simulink model "Projekt_Dyks_Jozwiak"  (R2013a)
settings: Solver=ode4  SolverMode=SingleTasking  StartTime=0.0  StopTime=30  FixedStep=0.01  RelTol=1e-3  AbsTol=1e-6
InitFcn:
  | mue = 0.0048847; % kg.m
  | J = 0.0016814; % kg.m2
  | g = 9.81; % m/s2
  | 
  | a = (mue*g)/J;
  | 
  | 
  | %%%%%%%%%%%%%% 1 %%
  | A1_1 = 0.2; f1_1 = 15;
  | A2_1 = 0.2; f2_1 = 10;
  | A3_1 = 0.2; f3_1 = 5;
  | %%%%%%%%%%%%%% 2 %%
  | A1_2 = 0.2; f1_2 = 4;
  | A2_2 = 0.2; f2_2 = 12;
  | A3_2 = 0.2; f3_2 = 20;
  | %%%%%%%%%%%%%% 3 %%
  | A1_3 = 0.2; f1_3 = 5;
  | A2_3 = 0.2; f2_3 = 8;
  | A3_3 = 0.2; f3_3 = 10;
  | %%%%%%%%%%%%%% 4 %%
  | A1_4 = 0.2; f1_4 = 20;
  | A2_4 = 0.2; f2_4 = 10;
  | A3_4 = 0.2; f3_4 = 5;
  | 
  | T1 = 0.2;
  | T2 = 0.1;
  | Tf = 0.05;
  | r = 0.1;
  | 
  | b0 = 1;
  | A = [0 1 0;
  |        0 0 1;
  |        0 0 0];
  | b_ = [0; b0; 0];
  | c = [1; 0; 0];
  | 
  | %% Liczenie k
  | w_CL = 5;
  | n=2;
  | k = zeros(n,1);
  | for i = 1:n
  |     k(i) = ((factorial(n))/(factorial(n-i+1)*factorial(i-1)))*w_CL^(n-i+1);
  | end
  | 
  | k_r = [k(2); 1];
  | 
  | %% Liczenie l
  | k_ESO = 50;
  | l = zeros(n+1,1);
  | 
  | for i = 1:n+1
  |     l(i) = (factorial(n+1)/(factorial(n-i+1)*factorial(i)))*(k_ESO)^(i);
  | end
  | 
  | %% W ARTYKULE MADONSKI K,L ODPOWIADA L I B W ARTYKULE JIN H.
  | l1 = k(2);
  | l2 = k(1);
  | 
  | B1 = l(1);
  | B2 = l(2);
  | B3 = l(3);
  | 
  | %% WYZNACZENIE PARAMETRÓW:
  | Kc = (B2 * l2 + B3 * l1)/(b0*(B1 * l1 + B2 + l2));
  | tau_i = (B2 * l2 + B3 * l1)/(B3 * l2);
  | tau_d = (B1 * l2 + B2 * l1 + B3)/(B2 * l2 + B3 * l1);
  | wl = sqrt(B1 * l1 + B2 + l2);
  | zeta_l = (B1 + l1)/(2*sqrt(B1 * l1 + B2 + l2));
  | %% Wzmocnienia regulatora CPID:
  | Kp = Kc;
  | Ki = Kc/tau_i;
  | Kd = Kc * tau_d;
undefined symbols (not defined in the file): RTDAC4PCIBaseAddress
libraries: simulink x2
settings Model: SimulationMode=external  ExtModeTrigDuration=50000  ExtModeTrigLevel=0.400000  Creator=jims  LastModifiedBy=Pracownik
settings DataIOCC: ExternalInput=[]  InitialState=[]  LimitDataPoints=off  MaxDataPoints=5000  SignalLoggingSaveFormat=ModelDataLogs  SaveOutput=off  SaveTime=off  SignalLoggingName=sigsOut
settings OptimizationCC: BooleanDataType=off  ExpressionDepthLimit=2147483647  InitFltsAndDblsToZero=on
settings DebuggingCC: SaveWithParameterizedLinksMsg=none  SignalResolutionControl=TryResolveAllWithWarning  SolverPrmCheckMsg=none  MultiTaskDSMMsg=warning  MultiTaskCondExecSysMsg=none  IntegerOverflowMsg=none  FcnCallInpInsideContextMsg=UseLocalSettings  StrictBusMsg=None
settings HardwareCC: ProdIntDivRoundTo=Zero  ProdEndianess=LittleEndian  ProdHWDeviceType=Generic->32-bit x86 compatible
settings RTWCC: SystemTargetFile=rtwin.tlc  TemplateMakefile=rtwin.tmf  Description=Real-Time Windows Target  ProcessScript=rtwin_make_rtw_hook  IncludeERTFirstTime=on  RTWCompilerOptimization=On
settings CodeAppCC: MaxIdLength=95
settings RTWinTargetCC: TargetLibSuffix=_rtwin.lib  TargetPreCompLibLocation=C:\Program Files\MATLAB\R2013a\toolbox\rtw\targets\rtwin\lib\win64  CodeReplacementLibrary=ANSI_C  RTWinDir=C:/PROGRA~1/MATLAB/R2013a/toolbox/rtw/targets/rtwin  TargetArch=win64

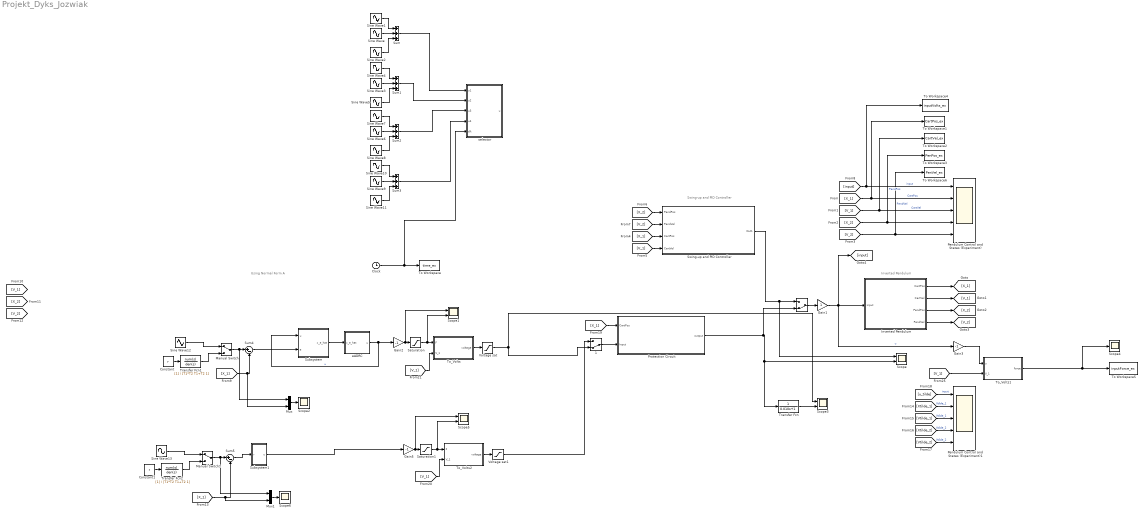
== system Projekt_Dyks_Jozwiak ==
  note: Using Normal Form A
  note: Inverted Pendulum
  note: Swing-up and PID Controller
  " " : ManualSwitch  CurrentSetting=0
  " 1" : ManualSwitch  CurrentSetting=0
  Clock : Clock
  Constant : Constant  Value=r
  Constant1 : Constant  Value=r
  Gain1 : Gain
  Gain2 : Gain  Gain=-1
  Gain3 : Gain  Gain=-1
  Gain5 : Gain  Gain=-1
  Inverted Pendulum : Subsystem
  Manual Switch : ManualSwitch
  Manual Switch1 : ManualSwitch
  Mux : Mux  Inputs=2
  Mux1 : Mux  Inputs=2
  Pendulum Control and States (Experiment) : Scope  NumInputPorts=5
      settings: TimeRange=7  YMin=-0.125~-0.125~-0.125~-3.5~-175000  YMax=0.15~0.125~0.125~3.5~175000  SaveName=P1_Data  MaxDataPoints=50000
  Pendulum Control and States (Experiment)1 : Scope  NumInputPorts=5
      settings: TimeRange=10  YMin=-1~-4~-7.5~-0.125~-0.25  YMax=1~4~7.5~0.075~0.2  SaveName=P1_Data1  MaxDataPoints=50000
  Protection Circuit : Subsystem
  Saturation : Saturate  UpperLimit=500  LowerLimit=-500
  Saturation1 : Saturate  UpperLimit=500  LowerLimit=-500
  Scope{,1,3,5} (4 alike) : Scope  NumInputPorts=2
      Scope settings: YMin=-5~-5  YMax=5~5
      Scope1 settings: YMin=-5~-5  YMax=5~5  SaveName=ScopeData2
      Scope3 settings: YMin=-0.3~-0.225  YMax=0.275~0.15  SaveName=ScopeData5
      Scope5 settings: YMin=-5~-5  YMax=5~5  SaveName=ScopeData6
  Scope2 : Scope
      settings: YMin=-0.11  YMax=0.11  SaveName=ScopeData3
  Scope4 : Scope
      settings: SaveName=ScopeData4
  Scope6 : Scope
      settings: YMin=-0.11  YMax=0.11  SaveName=ScopeData7
  Sine Wave : Sin  Amplitude=A2_1  Frequency=f2_1  SampleTime=0
  Sine Wave1 : Sin  Amplitude=A1_1  Frequency=f1_1  SampleTime=0
  Sine Wave10 : Sin  Amplitude=A1_4  Frequency=f1_4  SampleTime=0
  Sine Wave11 : Sin  Amplitude=A3_4  Frequency=f3_4  SampleTime=0
  Sine Wave12 : Sin  Amplitude=r  SampleTime=0
  Sine Wave13 : Sin  Amplitude=r  SampleTime=0
  Sine Wave2 : Sin  Amplitude=A3_1  Frequency=f3_1  SampleTime=0
  Sine Wave3 : Sin  Amplitude=A2_2  Frequency=f2_2  SampleTime=0
  Sine Wave4 : Sin  Amplitude=A1_2  Frequency=f1_2  SampleTime=0
  Sine Wave5 : Sin  Amplitude=A3_2  Frequency=f3_2  SampleTime=0
  Sine Wave6 : Sin  Amplitude=A2_3  Frequency=f2_3  SampleTime=0
  Sine Wave7 : Sin  Amplitude=A1_3  Frequency=f1_3  SampleTime=0
  Sine Wave8 : Sin  Amplitude=A3_3  Frequency=f3_3  SampleTime=0
  Sine Wave9 : Sin  Amplitude=A2_4  Frequency=f2_4  SampleTime=0
  Subsystem : Subsystem
  Subsystem1 : Subsystem
  Sum{,1..3} (4 alike) : Sum  Inputs=+++
  Sum4 : Sum  Inputs=|+-
  Sum5 : Sum  Inputs=|+-
  Swing-up and PID Controller : Subsystem
  To Workspace : ToWorkspace  VariableName=time_ex  SampleTime=-1
  To Workspace1 : ToWorkspace  VariableName=CartPos_ex  SampleTime=-1
  To Workspace2 : ToWorkspace  VariableName=CartVel_ex  SampleTime=-1
  To Workspace3 : ToWorkspace  VariableName=PenPos_ex  SampleTime=-1
  To Workspace4 : ToWorkspace  VariableName=inputVolts_ex  SampleTime=-1
  To Workspace5 : ToWorkspace  VariableName=inputForce_ex  SampleTime=-1
  To Workspace6 : ToWorkspace  VariableName=PenVel_ex  SampleTime=-1
  To_Volts : MATLAB Function  TreatAsAtomicUnit=on
  To_Volts1 : MATLAB Function  TreatAsAtomicUnit=on
  To_Volts2 : MATLAB Function  TreatAsAtomicUnit=on
  Transfer Fcn : TransferFcn  Denominator=[0.010 1]
  Transfer Fcn1 : TransferFcn  Denominator=[T1*T2 T1+T2 1]
  Transfer Fcn2 : TransferFcn  Denominator=[T1*T2 T1+T2 1]
  Voltage sat : Saturate  UpperLimit=0.6  LowerLimit=-0.6
  Voltage sat1 : Saturate  UpperLimit=0.6  LowerLimit=-0.6
  "eADRC " : Subsystem
  selector : MATLAB Function  TreatAsAtomicUnit=on
  wires:
  [V_2] -> To Workspace6/1, Pendulum Control and States (Experiment)/5  "PendVel"
  [X_2] -> To Workspace3/1, Pendulum Control and States (Experiment)/4  "PendPos"
  [V_1] -> To Workspace2/1, Pendulum Control and States (Experiment)/3  "CartVel"
  [X_1] -> To Workspace1/1, Pendulum Control and States (Experiment)/2  "CartPos"
  Inverted Pendulum/1(CartPos) -> [X_1]
  Inverted Pendulum/2(CartVel) -> [V_1]
  Inverted Pendulum/3(PendPos) -> [X_2]
  Inverted Pendulum/4(PendVel) -> [V_2]
  [X_2] -> Swing-up and PID Controller/1(PendPos)
  [V_2] -> Swing-up and PID Controller/2(PendVel)
  [X_1] -> Swing-up and PID Controller/3(CartPos)
  [V_1] -> Swing-up and PID Controller/4(CartVel)
  [input] -> To Workspace4/1, Pendulum Control and States (Experiment)/1  "input"
  Swing-up and PID Controller/1(Out1) -> Scope/1, " "/1
  "eADRC "/1("u ") -> Subsystem/1("u "), Gain2/1  "u"
  [Vtilde_2] -> Pendulum Control and States (Experiment)1/5  "Vtilde_2"
  [Xtilde_2] -> Pendulum Control and States (Experiment)1/4  "Xtilde_2"
  [Vtilde_1] -> Pendulum Control and States (Experiment)1/3  "Vtilde_1"
  [Xtilde_1] -> Pendulum Control and States (Experiment)1/2  "Xtilde_1"
  [u_tilde] -> Pendulum Control and States (Experiment)1/1  "input"
  Gain2/1 -> Saturation/1, Scope1/1
  [X_1] -> Protection Circuit/1(CartPos)
  Saturation/1 -> Scope1/2, To_Volts/1(F)
  [V_1] -> To_Volts/2(V_1)
  [X_1] -> Mux/2, Sum4/2
  " "/1 -> Gain1/1
  To_Volts/1(voltage) -> Voltage sat/1
  Transfer Fcn/1 -> Scope3/2
  Clock/1 -> selector/5(clk), To Workspace/1
  Protection Circuit/1(output) -> " "/2, Transfer Fcn/1, Scope/2
  Voltage sat/1 -> " 1"/2, Scope3/1
  " 1"/1 -> Protection Circuit/2(Input)
  Gain1/1 -> Gain3/1, Inverted Pendulum/1(input), [input]  "u"
  To_Volts1/1(force) -> Scope4/1, To Workspace5/1
  Gain3/1 -> To_Volts1/1(u)
  [V_1] -> To_Volts1/2(V_1)
  Sine Wave1/1 -> Sum/1
  Sine Wave/1 -> Sum/2
  Sine Wave2/1 -> Sum/3
  Sum/1 -> selector/1(u1)
  Sum1/1 -> selector/2(u2)
  Sum2/1 -> selector/3(u3)
  Sum3/1 -> selector/4(u4)
  Sine Wave4/1 -> Sum1/1
  Sine Wave3/1 -> Sum1/2
  Sine Wave5/1 -> Sum1/3
  Sine Wave7/1 -> Sum2/1
  Sine Wave6/1 -> Sum2/2
  Sine Wave8/1 -> Sum2/3
  Sine Wave10/1 -> Sum3/1
  Sine Wave9/1 -> Sum3/2
  Sine Wave11/1 -> Sum3/3
  Subsystem/1("x_e_hat ") -> "eADRC "/1("x_e_hat ")
  Constant/1 -> Transfer Fcn1/1
  Sine Wave12/1 -> Manual Switch/1
  Transfer Fcn1/1 -> Manual Switch/2
  Manual Switch/1 -> Mux/1, Sum4/1
  Sum4/1 -> Subsystem/2("e ")
  Mux/1 -> Scope2/1
  Constant1/1 -> Transfer Fcn2/1
  Sine Wave13/1 -> Manual Switch1/1
  Transfer Fcn2/1 -> Manual Switch1/2
  Manual Switch1/1 -> Mux1/1, Sum5/1
  Sum5/1 -> Subsystem1/1(r)
  [X_1] -> Mux1/2, Sum5/2
  Gain5/1 -> Saturation1/1, Scope5/1
  Saturation1/1 -> Scope5/2, To_Volts2/1(F)
  [V_1] -> To_Volts2/2(V_1)
  To_Volts2/1(voltage) -> Voltage sat1/1
  Subsystem1/1("u ") -> Gain5/1
  Voltage sat1/1 -> " 1"/1
  Mux1/1 -> Scope6/1

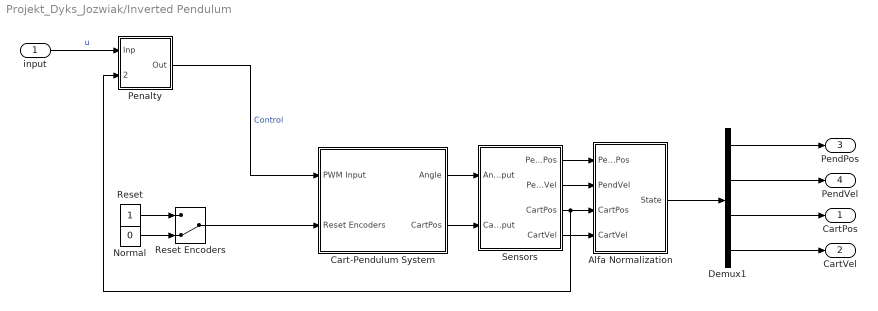
== system Projekt_Dyks_Jozwiak/Inverted Pendulum ==
  input : Inport
  Alfa Normalization : Subsystem  mask(Choose mode:){pos=Inverted Pendulum}
      mask prompts: pos "Choose mode:"
      mask TypeOptions pos: Inverted Pendulum | Crane Controller
  Cart-Pendulum System : Subsystem  mask{BaseAddress=RTDAC4PCIBaseAddress, T0=0.01}
      mask prompts: BaseAddress "Base Address:"; T0 "Sampling Period:"
      mask Display: plot( [0.725 0.725], [1.05 0.375], 0.725+0.05*sin([0:0.5:7]), 0.325+0.05*cos([0:0.5:7]), [-0.3 -0.3], [-0.3 -0.3], [1.8 1.8], [1.8 1.8], [0.1 1.4], [0.95 0.95], [0.1 1.4], [0.92 0.92], [0.65 0.8], [1 1], [0.65 0.8], [1.1 1.1], [0.65 0.65], [1.1 1], [0.8 0.8], [1 1.1] )
  Demux1 : Demux
  Normal : Constant  Value=0
  Penalty : Subsystem
  Reset : Constant
  Reset Encoders : ManualSwitch  CurrentSetting=0
  Sensors : Subsystem  mask(PENDULUM Output){T0=0.01}
      mask prompts: T0 "Sample Time"
      mask help: PCL-812 PG Device Driver
  CartPos : Outport
  CartVel : Outport  Port=2
  PendPos : Outport  Port=3
  PendVel : Outport  Port=4
  wires:
  Penalty/1(Out) -> Cart-Pendulum System/1(PWM Input)  "Control"
  Cart-Pendulum System/2(CartPos) -> Sensors/2(CartPosInput)
  Cart-Pendulum System/1(Angle) -> Sensors/1(AngleInput)
  Sensors/1(PendPos) -> Alfa Normalization/1(PendPos)
  Alfa Normalization/1(State) -> Demux1/1
  Sensors/2(PendVel) -> Alfa Normalization/2(PendVel)
  Reset/1 -> Reset Encoders/1
  Sensors/4(CartVel) -> Alfa Normalization/4(CartVel)
  Normal/1 -> Reset Encoders/2
  Reset Encoders/1 -> Cart-Pendulum System/2(Reset Encoders)
  Sensors/3(CartPos) -> Penalty/2(CartPos), Alfa Normalization/3(CartPos)
  Demux1/2 -> PendVel/1
  Demux1/1 -> PendPos/1
  Demux1/4 -> CartVel/1
  Demux1/3 -> CartPos/1
  input/1 -> Penalty/1(Inp)  "u"

== system Projekt_Dyks_Jozwiak/Protection Circuit ==
  CartPos : Inport
  Input : Inport  Port=2
  4 : Switch  SaturateOnIntegerOverflow=on  InputSameDT=on
  Rail limiter : MATLAB Function  TreatAsAtomicUnit=on
  Saturation1 : Saturate  UpperLimit=1  LowerLimit=-1
  Sign : Signum
  output : Outport
  wires:
  Rail limiter/1(logic) -> 4/2
  Sign/1 -> 4/1  "max"
  Input/1 -> 4/3
  CartPos/1 -> Rail limiter/1(CartPos), Sign/1
  4/1 -> Saturation1/1
  Saturation1/1 -> output/1

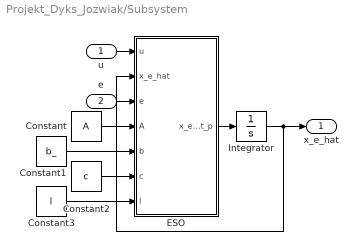
== system Projekt_Dyks_Jozwiak/Subsystem ==
  "u " : Inport
  "e " : Inport  Port=2
  Constant : Constant  Value=A
  Constant1 : Constant  Value=b_
  Constant2 : Constant  Value=c
  Constant3 : Constant  Value=l
  "ESO " : MATLAB Function  TreatAsAtomicUnit=on
  Integrator : Integrator  InitialCondition=[0; 0; 0]
  "x_e_hat " : Outport
  wires:
  Constant2/1 -> "ESO "/6(c)
  Constant/1 -> "ESO "/4(A)
  "ESO "/1(x_e_hat_p) -> Integrator/1
  Integrator/1 -> "x_e_hat "/1, "ESO "/2(x_e_hat)
  "u "/1 -> "ESO "/1(u)
  "e "/1 -> "ESO "/3(e)
  Constant3/1 -> "ESO "/7(l)
  Constant1/1 -> "ESO "/5(b)

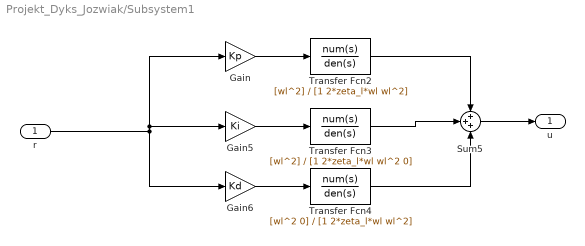
== system Projekt_Dyks_Jozwiak/Subsystem1 ==
  r : Inport
  Gain : Gain  Gain=Kp
  Gain5 : Gain  Gain=Ki
  Gain6 : Gain  Gain=Kd
  Sum5 : Sum  Inputs=+++
  Transfer Fcn2 : TransferFcn  Numerator=[wl^2]  Denominator=[1 2*zeta_l*wl wl^2]
  Transfer Fcn3 : TransferFcn  Numerator=[wl^2]  Denominator=[1 2*zeta_l*wl wl^2 0]
  Transfer Fcn4 : TransferFcn  Numerator=[wl^2 0]  Denominator=[1 2*zeta_l*wl wl^2]
  "u " : Outport
  wires:
  Transfer Fcn3/1 -> Sum5/2
  r/1 -> Gain/1, Gain5/1, Gain6/1
  Transfer Fcn4/1 -> Sum5/3
  Sum5/1 -> "u "/1
  Gain5/1 -> Transfer Fcn3/1
  Transfer Fcn2/1 -> Sum5/1
  Gain6/1 -> Transfer Fcn4/1
  Gain/1 -> Transfer Fcn2/1

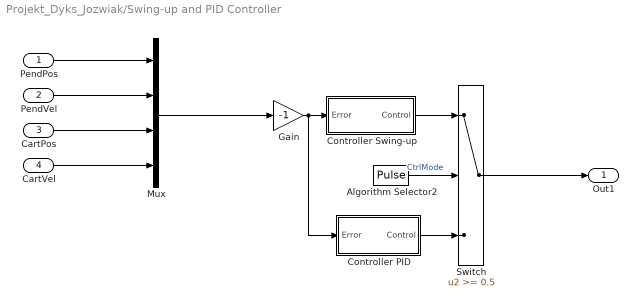
== system Projekt_Dyks_Jozwiak/Swing-up and PID Controller ==
  PendPos : Inport
  PendVel : Inport  Port=2
  CartPos : Inport  Port=3
  CartVel : Inport  Port=4
  Algorithm Selector2 : DiscretePulseGenerator  PulseType=Time based  Period=60  PulseWidth=85  SampleTime=0.01
  Controller PID : Subsystem  mask{Cart_PID=[ -0.8 -0.0 -0.05], Pend_PID=[-1 0 -0.0 ], Umax=0.5, zone=1.3, Friction=0.05, T0=0.01}
      mask prompts: Cart_PID "Cart PID parameters [Kp, Ki, Kd]:"; Pend_PID "Pendulum PID parameters [Kp, Ki, Kd]:"; Umax "Maximum control value:"; zone "Stabilisation zone [rad]:"; Friction "Friction compensation:"; T0 "Sample time:"
  Controller Swing-up : Subsystem
  Gain : Gain  Gain=-1
  Mux : Mux
  Switch : Switch  Threshold=0.5  SaturateOnIntegerOverflow=on  InputSameDT=on
  Out1 : Outport
  wires:
  Controller Swing-up/1(Control) -> Switch/1
  Algorithm Selector2/1 -> Switch/2  "CtrlMode"
  Gain/1 -> Controller Swing-up/1(Error), Controller PID/1(Error)
  Controller PID/1(Control) -> Switch/3
  Switch/1 -> Out1/1
  PendVel/1 -> Mux/2
  PendPos/1 -> Mux/1
  CartPos/1 -> Mux/3
  CartVel/1 -> Mux/4
  Mux/1 -> Gain/1

== system Projekt_Dyks_Jozwiak/eADRC  ==
  "x_e_hat " : Inport
  Constant : Constant  Value=b0
  Constant1 : Constant  Value=k
  MATLAB Function : MATLAB Function  TreatAsAtomicUnit=on
  "u " : Outport
  wires:
  Constant/1 -> MATLAB Function/1(b0)
  Constant1/1 -> MATLAB Function/2(k)
  MATLAB Function/1(u) -> "u "/1
  "x_e_hat "/1 -> MATLAB Function/3(x_e_hat)

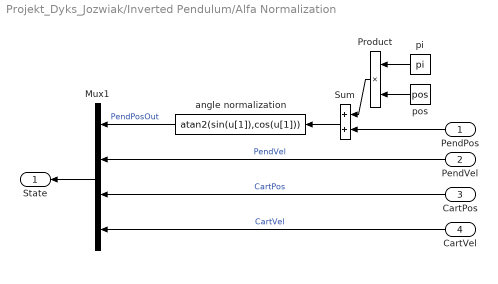
== system Projekt_Dyks_Jozwiak/Inverted Pendulum/Alfa Normalization ==
  PendPos : Inport
  PendVel : Inport  Port=2
  CartPos : Inport  Port=3
  CartVel : Inport  Port=4
  Mux1 : Mux
  Product : Product  SaturateOnIntegerOverflow=on  InputSameDT=on  OutDataTypeStr=Inherit: Same as first input
  Sum : Sum  SaturateOnIntegerOverflow=on  InputSameDT=on  OutDataTypeStr=Inherit: Same as first input
  angle normalization : Fcn  Expr=atan2(sin(u[1]),cos(u[1]))
  pi : Constant  Value=pi
  pos : Constant  Value=pos
  State : Outport  InitialOutput=0
  wires:
  angle normalization/1 -> Mux1/1  "PendPosOut"
  PendVel/1 -> Mux1/2  "PendVel"
  CartVel/1 -> Mux1/4  "CartVel"
  CartPos/1 -> Mux1/3  "CartPos"
  Mux1/1 -> State/1
  Sum/1 -> angle normalization/1
  PendPos/1 -> Sum/2
  pi/1 -> Product/1
  pos/1 -> Product/2
  Product/1 -> Sum/1

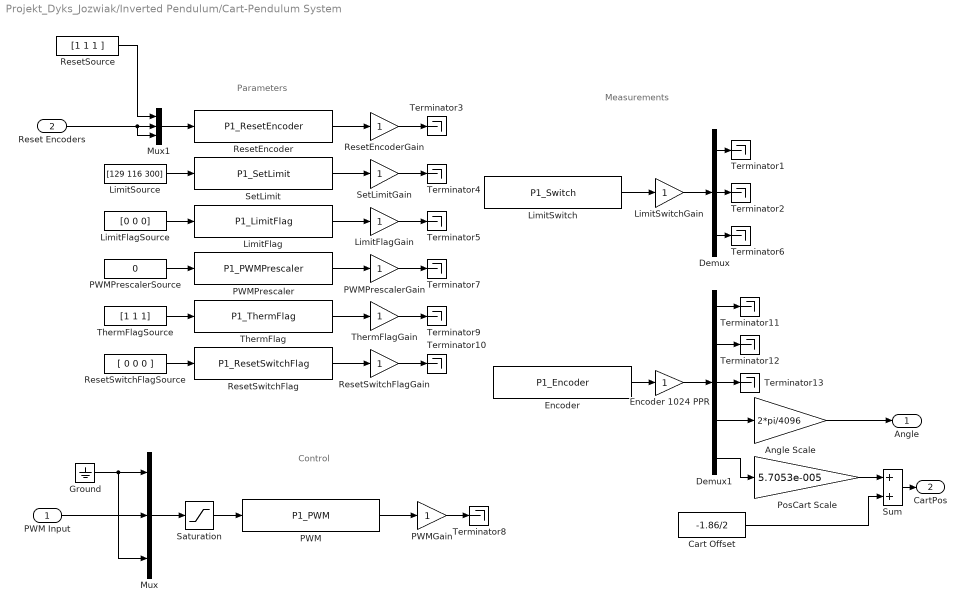
== system Projekt_Dyks_Jozwiak/Inverted Pendulum/Cart-Pendulum System ==
  note: Measurements
  note: Control
  note: Parameters
  PWM Input : Inport
  Reset Encoders : Inport  Port=2
  Angle Scale : Gain  Gain=2*pi/4096  OutDataTypeStr=Inherit: Same as input  ParamDataTypeStr=Inherit: Same as input
  Cart Offset : Constant  Value=-1.86/2
  Demux : Demux  Outputs=3
  Demux1 : Demux  Outputs=5
  Encoder : S-Function  FunctionName=P1_Encoder  Parameters=BaseAddress, T0  EnableBusSupport=off
  Encoder 1024 PPR : Gain  SaturateOnIntegerOverflow=on  OutDataTypeStr=Inherit: Same as input  ParamDataTypeStr=Inherit: Same as input
  Ground : Ground
  LimitFlag : S-Function  FunctionName=P1_LimitFlag  Parameters=BaseAddress, T0  EnableBusSupport=off
  LimitFlagGain : Gain  SaturateOnIntegerOverflow=on  OutDataTypeStr=Inherit: Same as input  ParamDataTypeStr=Inherit: Same as input
  LimitFlagSource : Constant  Value=[0 0 0]
  LimitSource : Constant  Value=[129 116 300]
  LimitSwitch : S-Function  FunctionName=P1_Switch  Parameters=BaseAddress, T0  EnableBusSupport=off
  LimitSwitchGain : Gain  SaturateOnIntegerOverflow=on  OutDataTypeStr=Inherit: Same as input  ParamDataTypeStr=Inherit: Same as input
  Mux : Mux  Inputs=3
  Mux1 : Mux  Inputs=[3 1 1]
  PWM : S-Function  FunctionName=P1_PWM  Parameters=BaseAddress, T0  EnableBusSupport=off
  PWMGain : Gain  SaturateOnIntegerOverflow=on  OutDataTypeStr=Inherit: Same as input  ParamDataTypeStr=Inherit: Same as input
  PWMPrescaler : S-Function  FunctionName=P1_PWMPrescaler  Parameters=BaseAddress, T0  EnableBusSupport=off
  PWMPrescalerGain : Gain  SaturateOnIntegerOverflow=on  OutDataTypeStr=Inherit: Same as input  ParamDataTypeStr=Inherit: Same as input
  PWMPrescalerSource : Constant  Value=0
  PosCart Scale : Gain  Gain=5.7053e-005  OutDataTypeStr=Inherit: Same as input  ParamDataTypeStr=Inherit: Same as input
  ResetEncoder : S-Function  FunctionName=P1_ResetEncoder  Parameters=BaseAddress, T0  EnableBusSupport=off
  ResetEncoderGain : Gain  SaturateOnIntegerOverflow=on  OutDataTypeStr=Inherit: Same as input  ParamDataTypeStr=Inherit: Same as input
  ResetSource : Constant  Value=[1 1 1 ]
  "ResetSwitchFlag " : S-Function  FunctionName=P1_ResetSwitchFlag  Parameters=BaseAddress, T0  EnableBusSupport=off
  ResetSwitchFlagGain : Gain  SaturateOnIntegerOverflow=on  OutDataTypeStr=Inherit: Same as input  ParamDataTypeStr=Inherit: Same as input
  ResetSwitchFlagSource : Constant  Value=[ 0 0 0 ]
  Saturation : Saturate  UpperLimit=1  LowerLimit=-1
  SetLimit : S-Function  FunctionName=P1_SetLimit  Parameters=BaseAddress, T0  EnableBusSupport=off
  SetLimitGain : Gain  SaturateOnIntegerOverflow=on  OutDataTypeStr=Inherit: Same as input  ParamDataTypeStr=Inherit: Same as input
  Sum : Sum  SaturateOnIntegerOverflow=on  InputSameDT=on  OutDataTypeStr=Inherit: Same as first input
  Terminator{1..13} (13 alike) : Terminator
  "ThermFlag " : S-Function  FunctionName=P1_ThermFlag  Parameters=BaseAddress, T0  EnableBusSupport=off
  ThermFlagGain : Gain  SaturateOnIntegerOverflow=on  OutDataTypeStr=Inherit: Same as input  ParamDataTypeStr=Inherit: Same as input
  ThermFlagSource : Constant  Value=[1 1 1]
  Angle : Outport
  CartPos : Outport  Port=2
  wires:
  Demux1/1 -> Terminator11/1
  Demux1/2 -> Terminator12/1
  Demux1/3 -> Terminator13/1
  Demux1/4 -> Angle Scale/1
  Demux1/5 -> PosCart Scale/1
  Angle Scale/1 -> Angle/1
  Demux/3 -> Terminator6/1
  Demux/2 -> Terminator2/1
  Demux/1 -> Terminator1/1
  LimitSwitchGain/1 -> Demux/1
  LimitSwitch/1 -> LimitSwitchGain/1
  Ground/1 -> Mux/1, Mux/3
  PWM Input/1 -> Mux/2
  ResetSwitchFlagGain/1 -> Terminator10/1
  ThermFlagGain/1 -> Terminator9/1
  PWMPrescalerGain/1 -> Terminator7/1
  LimitFlagGain/1 -> Terminator5/1
  SetLimitGain/1 -> Terminator4/1
  ResetEncoderGain/1 -> Terminator3/1
  ResetSwitchFlagSource/1 -> "ResetSwitchFlag "/1
  ThermFlagSource/1 -> "ThermFlag "/1
  PWMPrescalerSource/1 -> PWMPrescaler/1
  LimitFlagSource/1 -> LimitFlag/1
  LimitSource/1 -> SetLimit/1
  "ResetSwitchFlag "/1 -> ResetSwitchFlagGain/1
  "ThermFlag "/1 -> ThermFlagGain/1
  PWMPrescaler/1 -> PWMPrescalerGain/1
  LimitFlag/1 -> LimitFlagGain/1
  SetLimit/1 -> SetLimitGain/1
  ResetEncoder/1 -> ResetEncoderGain/1
  PWMGain/1 -> Terminator8/1
  PWM/1 -> PWMGain/1
  Mux/1 -> Saturation/1
  Saturation/1 -> PWM/1
  Encoder/1 -> Encoder 1024 PPR/1
  Encoder 1024 PPR/1 -> Demux1/1
  Mux1/1 -> ResetEncoder/1
  ResetSource/1 -> Mux1/1
  Reset Encoders/1 -> Mux1/2, Mux1/3
  PosCart Scale/1 -> Sum/1
  Sum/1 -> CartPos/1
  Cart Offset/1 -> Sum/2

== system Projekt_Dyks_Jozwiak/Inverted Pendulum/Penalty ==
  Inp : Inport
  CartPos : Inport  Port=2
  CtrlSat : Saturate  UpperLimit=1  LowerLimit=-1
  Fcn : Fcn  Expr=(u>=0.8)*(10*(u-0.8))^3 + (u<=-0.8)*(10*(u+0.8))^3
  Sum : Sum  Inputs=|++  SaturateOnIntegerOverflow=on  InputSameDT=on  OutDataTypeStr=Inherit: Same as first input
  Out : Outport
  wires:
  Inp/1 -> Out/1, Sum/1
  CartPos/1 -> Fcn/1
  Sum/1 -> CtrlSat/1
  Fcn/1 -> Sum/2

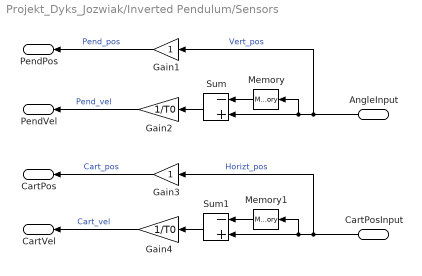
== system Projekt_Dyks_Jozwiak/Inverted Pendulum/Sensors ==
  AngleInput : Inport
  CartPosInput : Inport  Port=2
  Gain1 : Gain  SaturateOnIntegerOverflow=on  OutDataTypeStr=Inherit: Same as input  ParamDataTypeStr=Inherit: Same as input
  Gain2 : Gain  Gain=1/T0  SaturateOnIntegerOverflow=on  OutDataTypeStr=Inherit: Same as input  ParamDataTypeStr=Inherit: Same as input
  Gain3 : Gain  SaturateOnIntegerOverflow=on  OutDataTypeStr=Inherit: Same as input  ParamDataTypeStr=Inherit: Same as input
  Gain4 : Gain  Gain=1/T0  SaturateOnIntegerOverflow=on  OutDataTypeStr=Inherit: Same as input  ParamDataTypeStr=Inherit: Same as input
  Memory : Memory
  Memory1 : Memory
  Sum : Sum  Inputs=-+  SaturateOnIntegerOverflow=on  InputSameDT=on  OutDataTypeStr=Inherit: Same as first input
  Sum1 : Sum  Inputs=-+  SaturateOnIntegerOverflow=on  InputSameDT=on  OutDataTypeStr=Inherit: Same as first input
  PendPos : Outport  InitialOutput=0
  PendVel : Outport  Port=2  InitialOutput=0
  CartPos : Outport  Port=3  InitialOutput=0
  CartVel : Outport  Port=4  InitialOutput=0
  wires:
  Gain4/1 -> CartVel/1  "Cart_vel"
  Sum1/1 -> Gain4/1
  Memory1/1 -> Sum1/1
  Sum/1 -> Gain2/1
  Memory/1 -> Sum/1
  CartPosInput/1 -> Memory1/1, Sum1/2, Gain3/1  "Horizt_pos"
  AngleInput/1 -> Memory/1, Sum/2, Gain1/1  "Vert_pos"
  Gain2/1 -> PendVel/1  "Pend_vel"
  Gain1/1 -> PendPos/1  "Pend_pos"
  Gain3/1 -> CartPos/1  "Cart_pos"

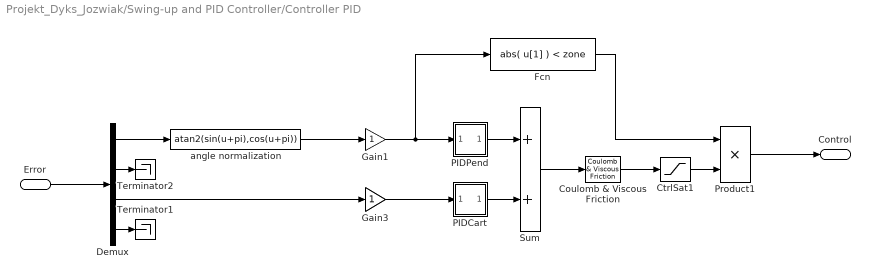
== system Projekt_Dyks_Jozwiak/Swing-up and PID Controller/Controller PID ==
  Error : Inport
  Coulomb & Viscous Friction : simulink/Discontinuities/Coulomb & Viscous Friction  offset=Friction  gain=1
  CtrlSat1 : Saturate  UpperLimit=Umax  LowerLimit=-Umax
  Demux : Demux
  Fcn : Fcn  Expr=abs( u[1] ) < zone
  Gain1 : Gain  SaturateOnIntegerOverflow=on  OutDataTypeStr=Inherit: Same as input  ParamDataTypeStr=Inherit: Same as input
  Gain3 : Gain  SaturateOnIntegerOverflow=on  OutDataTypeStr=Inherit: Same as input  ParamDataTypeStr=Inherit: Same as input
  PIDCart : Subsystem  mask(PID(2) Controller){P=Cart_PID(1), I=Cart_PID(2), D=Cart_PID(3), T0=T0}
      mask prompts: P "Proportional:"; I "Integral:"; D "Derivative:"; T0 "Sample Time:"
      mask help:
      | Enter Proportional(P), Integral(I), and Derivative(D) and divisor (N) terms.
      | P+I/s+Ds/(1/Ns+1)
      mask Help: This block implements a PID controller where parameters are entered for the Proportional, Integral and Derivative and divisor terms. Unmask this block to see how it works. The derivative term is implemented using an s/(s/N +1)  transfer function block. Making N large can create a "stiff" system.
      mask Display: disp('PID')
  PIDPend : Subsystem  mask(PID(2) Controller){P=Pend_PID(1), I=Pend_PID(2), D=Pend_PID(3), T0=T0}
      mask prompts: P "Proportional:"; I "Integral:"; D "Derivative:"; T0 "Sample Time:"
      mask help:
      | Enter Proportional(P), Integral(I), and Derivative(D) and divisor (N) terms.
      | P+I/s+Ds/(1/Ns+1)
      mask Help: This block implements a PID controller where parameters are entered for the Proportional, Integral and Derivative and divisor terms. Unmask this block to see how it works. The derivative term is implemented using an s/(s/N +1)  transfer function block. Making N large can create a "stiff" system.
      mask Display: disp('PID')
  Product1 : Product  SaturateOnIntegerOverflow=on  InputSameDT=on  OutDataTypeStr=Inherit: Same as first input
  Sum : Sum  SaturateOnIntegerOverflow=on  InputSameDT=on  OutDataTypeStr=Inherit: Same as first input
  Terminator1 : Terminator
  Terminator2 : Terminator
  angle normalization : Fcn  Expr=atan2(sin(u+pi),cos(u+pi))
  Control : Outport  InitialOutput=0
  wires:
  Demux/4 -> Terminator1/1
  Demux/3 -> Gain3/1
  Demux/2 -> Terminator2/1
  Error/1 -> Demux/1
  Demux/1 -> angle normalization/1
  Gain1/1 -> Fcn/1, PIDPend/1(In_1)
  PIDPend/1(Out_1) -> Sum/1
  Sum/1 -> Coulomb & Viscous Friction/1
  Coulomb & Viscous Friction/1 -> CtrlSat1/1
  CtrlSat1/1 -> Product1/2
  Fcn/1 -> Product1/1
  Product1/1 -> Control/1
  Gain3/1 -> PIDCart/1(In_1)
  PIDCart/1(Out_1) -> Sum/2
  angle normalization/1 -> Gain1/1

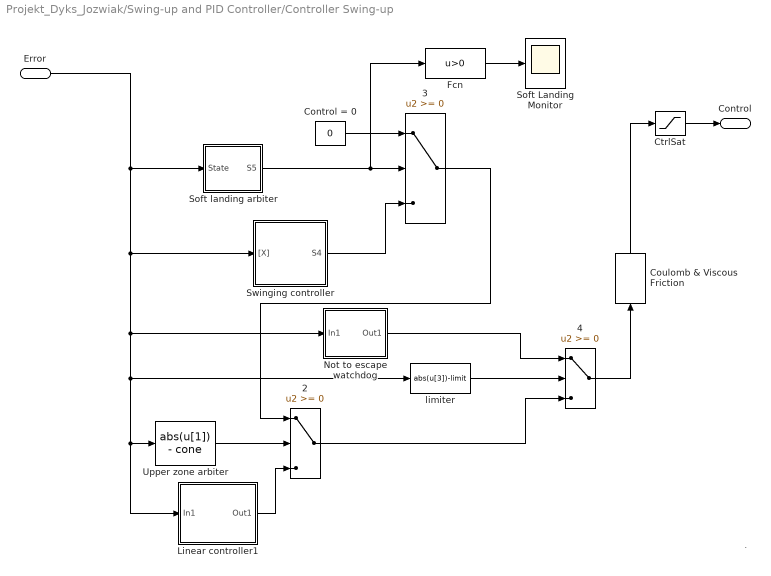
== system Projekt_Dyks_Jozwiak/Swing-up and PID Controller/Controller Swing-up ==
  note: .
  Error : Inport
  2 : Switch  SaturateOnIntegerOverflow=on  InputSameDT=on
  3 : Switch  SaturateOnIntegerOverflow=on  InputSameDT=on
  4 : Switch  SaturateOnIntegerOverflow=on  InputSameDT=on
  Control = 0 : Constant  Value=0
  Coulomb & Viscous Friction : simulink/Discontinuities/Coulomb & Viscous Friction  offset=0.001  gain=1
  CtrlSat : Saturate
  Fcn : Fcn  Expr=u>0
  Linear controller1 : Subsystem  mask(linear){umax1=0.2, K=[ 8 0.6 3.8 1.0 ]}
      mask prompts: umax1 "maximal control umax"; K "feedback K"
      mask Display: plot(0,0,100,100,[40,30,20],[87,85,80],[46,54,54,46,46],[90,90,80,80,90],[46,45,45,46,54,55,55,54,46],[78,80,90,91,91,90,80,78,78],[51,51,49,49],[78,10,10,78],[90,80,70,60],[70,80,85,88],[20,10],[80,70],[20,20,15],[73,80,80],[85,80,80],[80,80,74])
  Not to escape watchdog : Subsystem  mask{umax2=1}
      mask prompts: umax2 "maximal force"
      mask Display: plot(0,0,100,100,[20,40,40,20,20],[60,60,49,49,60],[56,59,40],[58,55,55],[56,59],[52,55],[38,13,13],[39,39,46],[46,13],[46,46],[23,23,24,22,24,24,22,23],[47,45,49,48,48,46,47,49],[36,35,34,34,37,34,36,35,36,37,35,34,35],[49,48,46,49,48,47,45,47,48,46,46,47,49],[22,22,24,24],[46,49,48,47])
  Soft Landing Monitor : Scope
      settings: TimeRange=60  YMin=0  YMax=1  MaxDataPoints=50000
  Soft landing arbiter : Subsystem  mask(Soft landing){k=8.5, R=0.3}
      mask prompts: k "k coefficient"; R "R value"
      mask help: Soft landing
      mask Display: plot(0,0,100,100,[14,20,20,14,14],[20,20,8,8,20],[40,35,35,40,40],[39,40,51,51,40],[60,55,55,56,60,60],[70,70,60,60,60,71],[74,74,80,80,74],[80,91,91,80,80])
  Swinging controller : Subsystem  mask(swing){umax=0.3}
      mask prompts: umax "maximal control umax"
      mask help: swing
      mask Display: plot(0,0,100,100,[20,20],[12,87],[93,90,90,93,7],[50,46,54,50,50],[20,22,18,20],[87,80,80,88],[80,80,75,75,71,71,65,65,60,60,49,49,40,40,20],[50,40,40,60,60,50,50,80,80,20,21,80,80,21,20])
  Upper zone arbiter : Fcn  Expr=abs(u[1]) - cone  mask(ZONE){cone=0.2}
      mask prompts: cone "width of stabilization zone [rad]"
      mask help: ZONE
      mask Display: plot(0,0,100,100,[40,60,80,83,80,60,40,20,17,20,40],[89,89,80,70,60,51,51,60,69,80,90],[83,50,17],[70,8,68])
  limiter : Fcn  Expr=abs(u[3])-limit  mask{limit=0.5}
      mask prompts: limit "rail limit"
      mask Display: plot(0,0,100,100,[10,90,90,10],[52,52,50,50],[30,30],[52,60],[70,68,68,70,70],[60,60,52,52,60],[30,32,32,30],[52,52,60,60])
  Control : Outport  InitialOutput=0
  wires:
  CtrlSat/1 -> Control/1
  Linear controller1/1(Out1) -> 2/3
  Upper zone arbiter/1 -> 2/2
  4/1 -> Coulomb & Viscous Friction/1
  Not to escape watchdog/1(Out1) -> 4/1
  limiter/1 -> 4/2
  Error/1 -> Not to escape watchdog/1(In1), Upper zone arbiter/1, Linear controller1/1(In1), limiter/1, Swinging controller/1("[X]"), Soft landing arbiter/1(State)
  Soft landing arbiter/1(S5) -> 3/2, Fcn/1
  Control = 0/1 -> 3/1
  Swinging controller/1(S4) -> 3/3
  3/1 -> 2/1
  2/1 -> 4/3
  Coulomb & Viscous Friction/1 -> CtrlSat/1
  Fcn/1 -> Soft Landing Monitor/1

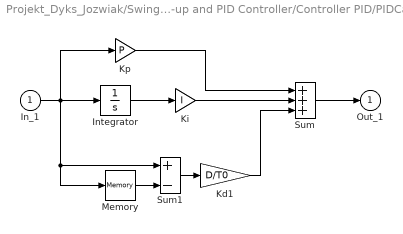
== system Projekt_Dyks_Jozwiak/Swing-up and PID Controller/Controller PID/PIDCart ==
  In_1 : Inport
  Integrator : Integrator  LimitOutput=on  UpperSaturationLimit=1  LowerSaturationLimit=-1
  Kd1 : Gain  Gain=D/T0  SaturateOnIntegerOverflow=on  OutDataTypeStr=Inherit: Same as input  ParamDataTypeStr=Inherit: Same as input
  Ki : Gain  Gain=I  SaturateOnIntegerOverflow=on  OutDataTypeStr=Inherit: Same as input  ParamDataTypeStr=Inherit: Same as input
  Kp : Gain  Gain=P  SaturateOnIntegerOverflow=on  OutDataTypeStr=Inherit: Same as input  ParamDataTypeStr=Inherit: Same as input
  Memory : Memory
  Sum : Sum  Inputs=+++  SaturateOnIntegerOverflow=on  InputSameDT=on  OutDataTypeStr=Inherit: Same as first input
  Sum1 : Sum  Inputs=+-  SaturateOnIntegerOverflow=on  InputSameDT=on  OutDataTypeStr=Inherit: Same as first input
  Out_1 : Outport  InitialOutput=0
  wires:
  Ki/1 -> Sum/2
  Integrator/1 -> Ki/1
  In_1/1 -> Integrator/1, Kp/1, Memory/1, Sum1/1
  Sum/1 -> Out_1/1
  Kp/1 -> Sum/1
  Memory/1 -> Sum1/2
  Sum1/1 -> Kd1/1
  Kd1/1 -> Sum/3

== system Projekt_Dyks_Jozwiak/Swing-up and PID Controller/Controller PID/PIDPend ==
  In_1 : Inport
  Integrator : Integrator  LimitOutput=on  UpperSaturationLimit=1  LowerSaturationLimit=-1
  Kd1 : Gain  Gain=D/T0  SaturateOnIntegerOverflow=on  OutDataTypeStr=Inherit: Same as input  ParamDataTypeStr=Inherit: Same as input
  Ki : Gain  Gain=I  SaturateOnIntegerOverflow=on  OutDataTypeStr=Inherit: Same as input  ParamDataTypeStr=Inherit: Same as input
  Kp : Gain  Gain=P  SaturateOnIntegerOverflow=on  OutDataTypeStr=Inherit: Same as input  ParamDataTypeStr=Inherit: Same as input
  Memory : Memory
  Sum : Sum  Inputs=+++  SaturateOnIntegerOverflow=on  InputSameDT=on  OutDataTypeStr=Inherit: Same as first input
  Sum1 : Sum  Inputs=+-  SaturateOnIntegerOverflow=on  InputSameDT=on  OutDataTypeStr=Inherit: Same as first input
  Out_1 : Outport  InitialOutput=0
  wires:
  Kd1/1 -> Sum/3
  Sum1/1 -> Kd1/1
  Memory/1 -> Sum1/2
  Kp/1 -> Sum/1
  Sum/1 -> Out_1/1
  In_1/1 -> Sum1/1, Memory/1, Kp/1, Integrator/1
  Integrator/1 -> Ki/1
  Ki/1 -> Sum/2

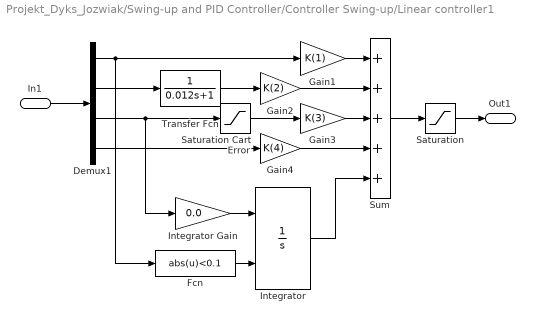
== system Projekt_Dyks_Jozwiak/Swing-up and PID Controller/Controller Swing-up/Linear controller1 ==
  In1 : Inport
  Demux1 : Demux
  Fcn : Fcn  Expr=abs(u)<0.1
  Gain1 : Gain  Gain=K(1)  SaturateOnIntegerOverflow=on  OutDataTypeStr=Inherit: Same as input  ParamDataTypeStr=Inherit: Same as input
  Gain2 : Gain  Gain=K(2)  SaturateOnIntegerOverflow=on  OutDataTypeStr=Inherit: Same as input  ParamDataTypeStr=Inherit: Same as input
  Gain3 : Gain  Gain=K(3)  SaturateOnIntegerOverflow=on  OutDataTypeStr=Inherit: Same as input  ParamDataTypeStr=Inherit: Same as input
  Gain4 : Gain  Gain=K(4)  SaturateOnIntegerOverflow=on  OutDataTypeStr=Inherit: Same as input  ParamDataTypeStr=Inherit: Same as input
  Integrator : Integrator  ExternalReset=rising  LimitOutput=on  UpperSaturationLimit=0.2  LowerSaturationLimit=-0.2
  Integrator Gain : Gain  Gain=0.0  SaturateOnIntegerOverflow=on  OutDataTypeStr=Inherit: Same as input  ParamDataTypeStr=Inherit: Same as input
  Saturation : Saturate  UpperLimit=umax1  LowerLimit=-umax1
  Saturation Cart Error : Saturate  UpperLimit=0.1  LowerLimit=-0.1
  Sum : Sum  Inputs=+++++  SaturateOnIntegerOverflow=on  InputSameDT=on  OutDataTypeStr=Inherit: Same as first input
  Transfer Fcn : TransferFcn  Denominator=[0.012 1]
  Out1 : Outport  InitialOutput=0
  wires:
  Saturation Cart Error/1 -> Gain3/1
  Integrator Gain/1 -> Integrator/1
  Fcn/1 -> Integrator/2
  Integrator/1 -> Sum/5
  Transfer Fcn/1 -> Gain2/1
  Demux1/1 -> Fcn/1, Gain1/1
  Saturation/1 -> Out1/1
  Gain1/1 -> Sum/1
  Gain2/1 -> Sum/2
  Demux1/2 -> Transfer Fcn/1
  Gain3/1 -> Sum/3
  Demux1/3 -> Saturation Cart Error/1, Integrator Gain/1
  Gain4/1 -> Sum/4
  Demux1/4 -> Gain4/1
  Sum/1 -> Saturation/1
  In1/1 -> Demux1/1

== system Projekt_Dyks_Jozwiak/Swing-up and PID Controller/Controller Swing-up/Not to escape watchdog ==
  In1 : Inport
  Fcn : Fcn  Expr=-u[3]
  Gain : Gain  Gain=umax2  SaturateOnIntegerOverflow=on  OutDataTypeStr=Inherit: Same as input  ParamDataTypeStr=Inherit: Same as input
  Sign : Signum
  Out1 : Outport  InitialOutput=0
  wires:
  In1/1 -> Fcn/1
  Fcn/1 -> Sign/1
  Gain/1 -> Out1/1
  Sign/1 -> Gain/1

== system Projekt_Dyks_Jozwiak/Swing-up and PID Controller/Controller Swing-up/Soft landing arbiter ==
  note: INPUT
  note: OUTPUT
  note: ENERGY CONTROL
  State : Inport
  Gain : Gain  Gain=9.81*k*R  SaturateOnIntegerOverflow=on  OutDataTypeStr=Inherit: Same as input  ParamDataTypeStr=Inherit: Same as input
  Kinetic Energy : Fcn  Expr=u[2]*u[2]*0.5
  Potential Energy : Fcn  Expr=cos(u[1])
  "one " : Constant
  s2 : Sum  SaturateOnIntegerOverflow=on  InputSameDT=on  OutDataTypeStr=Inherit: Same as first input
  s3 : Sum  Inputs=+-  SaturateOnIntegerOverflow=on  InputSameDT=on  OutDataTypeStr=Inherit: Same as first input
  S5 : Outport  InitialOutput=0
  wires:
  s2/1 -> S5/1
  State/1 -> Kinetic Energy/1, Potential Energy/1
  Gain/1 -> s2/2
  s3/1 -> Gain/1
  Kinetic Energy/1 -> s2/1
  "one "/1 -> s3/2
  Potential Energy/1 -> s3/1

== system Projekt_Dyks_Jozwiak/Swing-up and PID Controller/Controller Swing-up/Swinging controller ==
  "[X]" : Inport
  abs(x1) : Fcn  Expr=u[2]*(abs(u[1])-pi/2)
  swing : Relay  OffOutputValue=-1
  umax : Gain  Gain=umax  SaturateOnIntegerOverflow=on  OutDataTypeStr=Inherit: Same as input  ParamDataTypeStr=Inherit: Same as input
  S4 : Outport  InitialOutput=0
  wires:
  abs(x1)/1 -> swing/1
  swing/1 -> umax/1
  "[X]"/1 -> abs(x1)/1
  umax/1 -> S4/1

== matlab function Projekt_Dyks_Jozwiak/To_Volts ==
  data: F input; voltage output; V_1 input
function voltage = To_Volts(F,V_1)

p1 = 9.4;
p2 = -0.548;

voltage = (F - p2*V_1)/p1;

== matlab function Projekt_Dyks_Jozwiak/eADRC /MATLAB Function ==
  data: u output; b0 input; k input; x_e_hat input
function u = fcn(b0, k, x_e_hat)

k = k';
kpom = [k, 1];
b0_1 = 1/b0;
u = b0_1*(kpom*x_e_hat);

== matlab function Projekt_Dyks_Jozwiak/Subsystem/ESO  ==
  data: u input; x_e_hat input; e input; A input; b input; c input; l input; x_e_hat_p output
function x_e_hat_p = fcn(u, x_e_hat, e, A, b, c, l)
c = c';
pom1 = c*x_e_hat;
pom2 = e - pom1;

x_e_hat_p1 = A*x_e_hat-b*u+l*pom2;
x_e_hat_p = x_e_hat_p1(:,1);

== matlab function Projekt_Dyks_Jozwiak/To_Volts2 ==
  data: F input; voltage output; V_1 input
function voltage = To_Volts(F,V_1)

p1 = 9.4;
p2 = -0.548;

voltage = (F - p2*V_1)/p1;

== matlab function Projekt_Dyks_Jozwiak/Protection Circuit/Rail limiter ==
  data: CartPos input; logic output
function logic = Condition(CartPos)

logic = -1;
con = 0.7;

if (CartPos >= con ) || (CartPos <= -con)
        logic = 1;
end


end

== matlab function Projekt_Dyks_Jozwiak/To_Volts1 ==
  data: u input; force output; V_1 input
function force = To_Force(u,V_1)

p1 = 9.4;
p2 = -0.548;

force = p1*u + p2*V_1;

== matlab function Projekt_Dyks_Jozwiak/selector ==
  data: u1 input; u output; u2 input; u3 input; u4 input; clk input
function u = selector(u1,u2,u3,u4,clk)

u=0;

if clk >= 0 && clk < 3
    u = u1;
elseif clk >= 3 && clk < 6
    u = u2;
elseif clk >= 6 && clk < 9
    u = u3;
elseif clk >= 9 && clk < 12
    u = u4;
end


end
